simulink model "sim_nomal_regulator"  (R2019a)
settings: Solver=FixedStepAuto  StartTime=0.0  StopTime=20  FixedStep=sT  RelTol=1e-3
InitFcn:
  | sim_param;
values from neighbouring files (symbols this model uses):
  bn = 50    [robot_param.m]    (also in sim_robot_param.m)
  bt = 50    [robot_param.m]    (also in sim_robot_param.m)
  foot_x = 0.07    [robot_param.m]    (also in sim_robot_param.m)
  foot_y = 0.045    [robot_param.m]    (also in sim_robot_param.m)
  foot_z = 0.01    [robot_param.m]    (also in sim_robot_param.m)
  height_plane = 0.025    [robot_param.m]    (also in sim_robot_param.m)
  inix = [0.00 0.00]'    [param.m]    (also in sim_param.m)
  iniXzmax = 0.05    [param.m]    (also in sim_param.m)
  iniXzmin = -0.05    [param.m]    (also in sim_param.m)
  iniy = [0.00 0.00]'    [param.m]    (also in sim_param.m)
  iniYzmax = 0.0625    [param.m]    (also in sim_param.m)
  iniYzmin = -0.0625    [param.m]    (also in sim_param.m)
  kn = 5000    [robot_param.m]    (also in sim_robot_param.m)
  kt = 5000    [robot_param.m]    (also in sim_robot_param.m)
  mu_d = 0.8    [robot_param.m]    (also in sim_robot_param.m)
  mu_s = 2    [robot_param.m]    (also in sim_robot_param.m)
  plane_x = 3    [robot_param.m]    (also in sim_robot_param.m = 6)
  plane_y = 1    [robot_param.m]    (also in sim_robot_param.m)
  R = 20    [param.m]    (also in sim_param.m = 1)
  sT = 0.02    [param.m]    (also in sim_param.m = 0.001)
  torso_offset_x = 0.0    (= 0)    [robot_param.m]    (also in sim_robot_param.m)
  torso_offset_z = -torso_z/2    (= -0.05)    [robot_param.m]    (also in sim_robot_param.m)
  torso_x = 0.1    [robot_param.m]    (also in sim_robot_param.m)
  torso_y = 0.08    [robot_param.m]    (also in sim_robot_param.m)
  torso_z = 0.10    (= 0.1)    [robot_param.m]    (also in sim_robot_param.m)
  w = sqrt(g/zc)    [param.m]    (also in sim_param.m)
  zvt = 1e-3    (= 0.001)    [robot_param.m]    (also in sim_robot_param.m)
undefined symbols (not defined in the file or in its folder): Ad, Bd, Cd, Dd, DiscIntNeverNeededParam, Discrete, sigbuilder_block, Time, X, Y, Z
libraries: nesl_utility x142, sm_lib x86, cstblocks x11, ctrlSharedLib x8
(part 6 of 6)

== stateflow chart sim_nomal_regulator/simulation/Robot/Right Leg/Subsystem4/Chart ==
  state No_Contact/
    (default) -> (junction 3) : {
        | mode = 1;
        |
        | Fn = 0;
        | Fx = 0; Fy = 0;
        | }
  state Sticking
    Sticking -> (junction 35) [order 1] : {
        | Fn = -(kn*pn+bn*dpn);
        | }
    (default) -> (junction 33) : {
        | mode = 4;
        |
        | Fn = -(kn*pn+bn*dpn);
        | }
    (junction 33) -> (junction 35)
    (junction 35) -> (junction 36) [order 1] : [Fn < 0]
    (junction 35) -> (junction 37) [order 2] : {
        | Fx = -(kt*(px-ax)+bt*dpx);
        | Fy = -(kt*(py-ay)+bt*dpy);
        |
        | norm_Ft = sqrt(Fx^2+Fy^2);
        | }
    (junction 36) -> (junction 41) : {
        | mode = 6;
        |
        | Fn = 0;
        | Fx = 0; Fy = 0;
        | }
    (junction 37) -> (junction 40) [order 1] : [norm_Ft > mu_s*Fn]
    (junction 37) -> (junction 38) [order 2]
    (junction 40) -> (junction 42) : {
        | mode = 5;
        |
        | Fx = mu_s*Fn*Fx/norm_Ft;
        | Fy = mu_s*Fn*Fy/norm_Ft;
        | }
    (junction 42) -> (junction 38)
    (junction 41) -> (junction 42)
    (junction 38) -> (junction 39)
  state Sliding
    Sliding -> (junction 10) [order 1] : {
        | mode = 2;
        |
        | Fn = -(kn*pn+bn*dpn);
        | }
    (default) -> (junction 8) : {
        | mode = 2;
        |
        | Fn = -(kn*pn+bn*dpn);
        | }
    (junction 8) -> (junction 10)
    (junction 10) -> (junction 11) [order 1] : [Fn < 0]
    (junction 10) -> (junction 12) [order 2] : {
        | norm_dpt = sqrt(dpx^2+dpy^2);
        | }
    (junction 11) -> (junction 17) : {
        | mode = 6;
        |
        | Fn = 0;
        | Fx = 0; Fy = 0;
        | }
    (junction 12) -> (junction 15) [order 1] : [norm_dpt <= zvt]
    (junction 12) -> (junction 13) [order 2] : {
        | Fx = -mu_d*Fn*dpx/norm_dpt;
        | Fy = -mu_d*Fn*dpy/norm_dpt;
        | }
    (junction 15) -> (junction 16) : {
        | mode = 3;
        | Fx = -mu_d*Fn*dpx/zvt;
        | Fy = -mu_d*Fn*dpy/zvt;
        |
        | ax = px;
        | ay = py;
        | }
    (junction 16) -> (junction 13)
    (junction 17) -> (junction 16)
    (junction 13) -> (junction 14)
  (default) -> No_Contact
  No_Contact -> Sliding : [pn < 0]
  Sliding -> No_Contact [order 1] : [pn >= 0]
  Sticking -> No_Contact [order 1] : [pn >= 0]
  Sliding -> Sticking [order 2] : [pn < 0 ...
      | && mode == 3]
  Sticking -> Sliding [order 2] : [pn < 0 ...
      | && (mode == 5 || mode == 6)]
  data: kn input; kt input; Fx output double; Fy output double; ax local double; ay local double; bn input; bt input; mu_d input; mu_s input; zvt input; px input; py input; pn input; dpx input; dpy input; dpn input; norm_Ft local double; norm_dpt local double; Fn output double; mode output double

== matlab function sim_nomal_regulator/calcULINK ==
  settings: updateMethod=DISCRETE
  data: sT input; u input; sys output; uLINK data_store_memory
function sys = calcULINK(sT,u)

    %u[腰X 腰Y 右足X 右足Y 右足Z 左足X 左足Y 左足Z]

    global uLINK;
    
    persistent cnt;
    if isempty(cnt)
        cnt = 0.0;
    end
    
    ToDeg = 180/pi;
    ToRad = pi/180;
    
    sys = zeros(12,1);
    
    %%% ZMPの計算
    %com = calcCoM;  % 重心位置
    %P = calcP(1);   % 並進運動量
    %L = calcL(1);   % 原点回りの角運動量
    
    %Zc  = com(3);      % 線形倒立振子の設定高さ
    %Tc  = sqrt(Zc/G);  % 線形倒立振子の時定数
    %cx0 = com(1);
    %cy0 = com(2);
    
    
    p0 = uLINK(JointName.BODY).p;
    uLINK(JointName.BODY).p = [u(1), u(2), uLINK(JointName.BODY).p(3)]';
    v = (uLINK(JointName.BODY).p-p0)/sT;
    uLINK(JointName.BODY).v = [v(1) v(2) v(3)]';
    uLINK(JointName.BODY).R = RPY2R([0 0*ToRad 0]);

    %ForwardKinematics(1);
    
    p = [u(3) u(4) u(5)]';
    Rfoot.p = [u(3) u(4) u(5)]';
    Rfoot.R = RPY2R([0 0 0]);
    v = (p-uLINK(JointName.RLEG_FOOT).p)/sT;
    Rfoot.v = [v(1) v(2) v(3)]';
    Rfoot.w = [0 0 0]';
    InverseKinematicsAll(8, Rfoot);
    
    p = [u(6) u(7) u(8)]';
    Lfoot.p = [u(6) u(7) u(8)]';
    Lfoot.R = RPY2R([0 0 0]);
    v = (p-uLINK(JointName.LLEG_FOOT).p)/sT;
    Lfoot.v = [v(1) v(2) v(3)]';
    Lfoot.w = [0 0 0]';
    InverseKinematicsAll(15, Lfoot);
    
    ForwardVelocity(1); 
    
    
    %{
    sys = [90 90 90 90 90 90 90 90 90 90 90 90]';
    
    sys(1) = round(rad2deg(uLINK(JointName.RLEG_J0).q))+90;
    %股関節の剛性不足による胴体の傾き補償フィードフォワード
    sys(2) = round(rad2deg(uLINK(JointName.RLEG_J1).q))+90-0;
    sys(3) = -round(rad2deg(uLINK(JointName.RLEG_J2).q))+90;
    sys(4) = -round(rad2deg(uLINK(JointName.RLEG_J3).q))+90;
    sys(5) = -round(rad2deg(uLINK(JointName.RLEG_J4).q))+90;
    sys(6) = -round(rad2deg(uLINK(JointName.RLEG_J5).q))+90;
    
    sys(7) = round(rad2deg(uLINK(JointName.LLEG_J0).q))+90;
    sys(8) = round(rad2deg(uLINK(JointName.LLEG_J1).q))+90+0;
    sys(9) = -round(rad2deg(uLINK(JointName.LLEG_J2).q))+90;
    sys(10) = -round(rad2deg(uLINK(JointName.LLEG_J3).q))+90;
    sys(11) = -round(rad2deg(uLINK(JointName.LLEG_J4).q))+90;
    sys(12) = -round(rad2deg(uLINK(JointName.LLEG_J5).q))+90;
    %}
    sys(1) = uLINK(JointName.RLEG_J0).q;
    sys(2) = uLINK(JointName.RLEG_J1).q-deg2rad(0);
    sys(3) = uLINK(JointName.RLEG_J2).q;
    sys(4) = uLINK(JointName.RLEG_J3).q;
    sys(5) = uLINK(JointName.RLEG_J4).q;
    sys(6) = uLINK(JointName.RLEG_J5).q;
    sys(7) = uLINK(JointName.LLEG_J0).q;
    sys(8) = uLINK(JointName.LLEG_J1).q+deg2rad(0);
    sys(9) = uLINK(JointName.LLEG_J2).q;
    sys(10) = uLINK(JointName.LLEG_J3).q;
    sys(11) = uLINK(JointName.LLEG_J4).q;
    sys(12) = uLINK(JointName.LLEG_J5).q;
    
    cnt = cnt + sT;
end

== matlab function sim_nomal_regulator/MATLAB Function3 ==
  data: x output; sT input
function x = orbit(sT)

    persistent t; 
    if (isempty(t))     
        t = 0;
    end
    
    %x = zeros(3,1);
    %x = create_orbit(t, 0, 0.6, 0.1);
    x = create_orbit(t, 0, 1.8, 0.3);
    %x = create_orbit(t, 0, 3.0, 0.5);
    
    %{
    x = zeros(3,1);
    if (t > 2)
        x = [0 0.5 0]';
    end
    %}
    t = t + sT;
end

%% 
%
% t:現在時間
% eta0:初期位置
% eta3:最終位置
% d_eta1:最高速度
function Y = create_orbit(t, eta0, eta3, d_eta1)

    %最高速度
    %d_eta1 = 0.1;

    %初期時間
    t0 = 2;
    %加速終了時間（等速度開始時間）
    t1 = 4;
    %等速度終了時間（減速開始時間）
    t2 = 8;
    %減速終了時間
    t3 = 10;


    %加速終了時の位置
    eta1 = eta0 + (d_eta1*(t1-t0)/2);
    %等速終了時の位置
    eta2 = eta1 + (d_eta1*(t2-t1));

    ETA1 = [eta0 0 0 eta1 d_eta1 0]';
    ETA3 = [eta2 d_eta1 0 eta3 0 0]';

    H = [t0^5 t0^4 t0^3 t0^2 t0 1;
        5*t0^4 4*t0^3 3*t0^2 2*t0 1 0;
        20*t0^3 12*t0^2 6*t0 2 0 0;
        t1^5 t1^4 t1^3 t1^2 t1 1;
        5*t1^4 4*t1^3 3*t1^2 2*t1 1 0;
        20*t1^3 12*t1^2 6*t1 2 0 0];
    A = H\ETA1;

    H = [t2^5 t2^4 t2^3 t2^2 t2 1;
        5*t2^4 4*t2^3 3*t2^2 2*t2 1 0;
        20*t2^3 12*t2^2 6*t2 2 0 0;
        t3^5 t3^4 t3^3 t3^2 t3 1;
        5*t3^4 4*t3^3 3*t3^2 2*t3 1 0;
        20*t3^3 12*t3^2 6*t3 2 0 0];
    B = H\ETA3;


    Y = zeros(3,1);
    if (t < t0) 
        Y(1) = eta0;
        Y(2) = 0;
        Y(3) = 0;
    %加速
    elseif (t0 <= t && t < t1) 
        Y(1) = A(1)*t^5 + A(2)*t^4 + A(3)*t^3 + A(4)*t^2 + A(5)*t + A(6);
        Y(2) = 5*A(1)*t^4 + 4*A(2)*t^3 + 3*A(3)*t^2 + 2*A(4)*t + A(5);
        Y(3) = 20*A(1)*t^3 + 12*A(2)*t^2 + 6*A(3)*t + 2*A(4);
    %等速
    elseif (t1 <= t && t <= t2)
        Y(1) = (t-t1)*d_eta1 + eta1;
        Y(2) = d_eta1;
        Y(3) = 0;
    %減速
    elseif (t2 < t && t <= t3)
        Y(1) = B(1)*t^5 + B(2)*t^4 + B(3)*t^3 + B(4)*t^2 + B(5)*t + B(6);
        Y(2) = 5*B(1)*t^4 + 4*B(2)*t^3 + 3*B(3)*t^2 + 2*B(4)*t + B(5);
        Y(3) = 20*B(1)*t^3 + 12*B(2)*t^2 + 6*B(3)*t + 2*B(4);
    else
        Y(1) = eta3;
        Y(2) = 0;
        Y(3) = 0;
    end


end

== matlab function sim_nomal_regulator/regulator1/MATLAB Function ==
  data: refZmp output; xzArea output; yzArea output; x input; legR output; legL output; y input; w input; iniXzmax input; iniXzmin input; iniYzmax input; iniYzmin input; refVx input
function [refZmp,xzArea,yzArea,legR,legL] = fcn(x,y,w,iniXzmax,iniXzmin,iniYzmax,iniYzmin,refVx)
    
    
    %% x軸
    qx = 0.5;
    persistent xR;
    if isempty(xR)
        xR = 0.0;
    end
    persistent xL;
    if isempty(xL)
        xL = 0.0;
    end
    
    %% y軸
    qy = 0.5;
    %r 振幅
    r = 0.05;
    k = 1;
    persistent rho;
    if isempty(rho)
        rho = 1;
    end
    
    %% z軸
    %左足裏内側縁
    xLin = 0.0175;
    %右足裏内側縁
    xRin = -0.0175;
    
    %% y軸
    refy = 0.0;
    zeta = sqrt( (y(1)-refy)^2 + (y(2)^2/(w^2*qy)) );
    f = 1-rho*exp( k*(1-((qy+1)^2*zeta^2)/r^2) );
    yz = refy+(qy+1)*(y(1)-refy + f*(y(2)/w));
    
    yzmax = iniYzmax;
    yzmin = iniYzmin;
    Yz = yz -refy;
    
    %% z軸   
    %右足高さ
    zR = clac(Yz,y,w,rho,xLin,r);
    if (zR > 0) 
        yzmin = refy + xLin;
    end
    %左足高さ
    zL = clac(Yz,y,w,rho,xRin,r);
    if (zL > 0) 
        yzmax = refy + xRin;
    end
    
    if (yz > yzmax)
        yz = yzmax;
    elseif (yz < yzmin)
        yz = yzmin;
    end
    
    refys = y(1)+(y(2)/w);
    yR = -0.04;
    yL = 0.04;
    
    %% x軸
    refx = x(1);
    if (refVx == 0) 
        %立位可安定
        qx = 1.0;
    else
        %速度追従
        qx = 0.0;
    end
    
    %ZMP
    xz = refx+(qx+1)*(x(1)-refx + (x(2)-refVx)/w);
    %着地位置
    refxs = x(1)+(x(2)/w);
    
    if (zR > 0)
        xR = refxs;
        xzmax = xL + iniXzmax;
        xzmin = xL + iniXzmin;
    elseif (zL > 0)
        xL = refxs;
        xzmax = xR + iniXzmax;
        xzmin = xR + iniXzmin;
    else
        if (xL > xR)
            xzmax = xL + iniXzmax;
            xzmin = xR + iniXzmin;
        else
            xzmax = xR + iniXzmax;
            xzmin = xL + iniXzmin;
        end
    end
    
    if (xz > xzmax)
        xz = xzmax;
    elseif (xz < xzmin)
        xz = xzmin;
    end
    
    refZmp = zeros(2,1);
    refZmp = [xz yz]';
    %refZmp = [0 0]';
    xzArea = [xzmax xzmin]';
    yzArea = [yzmax yzmin]';
    
    legR = [xR yR zR]';
    legL = [xL yL zL]';
   
    
end

%% 
function z = clac(yz,x,w,rho,xLin,r)
    
    q = 0.5;
    h = 0.02;
     
    pz = yz - ((q+1)*x(2)/w*sqrt(q))*1i;
    
    %軸足内側に入った
    pLin = xLin - sqrt(complex(abs(pz)^2-xLin^2))*1i;
    %軸足内側から出た
    pLout = xLin + sqrt(complex(abs(pz)^2-xLin^2))*1i;
    
    z = 0;
    phiL = 0;
    %左が軸足
    if (xLin > 0)
        %ZMPが左足にある
        if (real(pz) > xLin)
            %plinからpzまでの角度
            ang_pz = angle(pz)-angle(pLin);
            %pLinからpLoutまでの角度
            ang_io = angle(pLout)-angle(pLin);
            phiL = ang_pz/ang_io;
        end
    %右が軸足
    else
        %ZMPが右足にある
        if (real(pz) < xLin)
            %plinからpzまでの角度（負なので正（第一、第二象限）に移す）
            ang_pz = 0;
            if (angle(pz) > 0) 
                ang_pz = angle(pz)-pi+angle(pLin)+pi; 
            else
                ang_pz = angle(pz)+pi+angle(pLin)+pi; 
            end
            %pLinからpLoutまでの角度（負なので正（第一、第二象限）に移す）
            ang_io = angle(pLin)+pi-angle(pLout)+pi;
            phiL = ang_pz/ang_io;
        end
    end
    
    if (0 < phiL && phiL < 1)
        z = (1/2)*(h*abs(pz)/r)*sigma(rho)*(1-cos(2*pi*phiL));
    end
end

function y = sigma(rho)
    
    if (rho > 1)
        y = 1;
    elseif (exp(-1) <= rho && rho <= 1)
        y = (rho-exp(-1))/(1-exp(-1));
    else
        y = 0;
    end
end

== matlab function sim_nomal_regulator/MATLAB Function1 ==
  settings: updateMethod=DISCRETE
  data: u input; px output; py output; rx input; lx input
function [px,py] = fcn(u,rx,lx)
    
    r = -0.04;
    l = 0.04;
    xs = 0.07/2;
    ys = 0.045/2;
    
    
    r1x = (rx+xs)*u(1);
    r2x = (rx+xs)*u(2);
    r3x = (rx-xs)*u(3);
    r4x = (rx-xs)*u(4);
    PrxfRz = r1x+r2x+r3x+r4x;
    
    r1y = (r+ys)*u(1);
    r2y = (r-ys)*u(2);
    r3y = (r+ys)*u(3);
    r4y = (r-ys)*u(4);
    PryfRz = r1y+r2y+r3y+r4y;
    
    l1x = (lx+xs)*u(5);
    l2x = (lx+xs)*u(6);
    l3x = (lx-xs)*u(7);
    l4x = (lx-xs)*u(8);
    PlxfLz = l1x+l2x+l3x+l4x;
    
    l1y = (l+ys)*u(5);
    l2y = (l-ys)*u(6);
    l3y = (l+ys)*u(7);
    l4y = (l-ys)*u(8);
    PlyfLz = l1y+l2y+l3y+l4y;
    
    fRz = u(1)+u(2)+u(3)+u(4);
    fLz = u(5)+u(6)+u(7)+u(8);
    
    %両足が浮いてない
    if (fRz+fLz ~= 0) 
        %x軸のずれ0.02加算
        px = (PrxfRz+PlxfLz)/(fRz+fLz)+0.02;
        py = (PryfRz+PlyfLz)/(fRz+fLz);
    else
        px = 0;
        py = 0;
    end
    
    %{
    FnR_FrontLeft
    FnR_FrontRight
    FnR_RearLeft
    FnR_RearRight
    
    
    FnL_FrontLeft
    FnL_FrontRight
    FnL_RearLeft
    FnL_RearRight
    %}
    
    
end

== stateflow chart sim_nomal_regulator/simulation/Robot/Right Leg/Subsystem7/Chart ==
  state No_Contact/
    (default) -> (junction 3) : {
        | mode = 1;
        |
        | Fn = 0;
        | Fx = 0; Fy = 0;
        | }
  state Sticking
    Sticking -> (junction 35) [order 1] : {
        | Fn = -(kn*pn+bn*dpn);
        | }
    (default) -> (junction 33) : {
        | mode = 4;
        |
        | Fn = -(kn*pn+bn*dpn);
        | }
    (junction 33) -> (junction 35)
    (junction 35) -> (junction 36) [order 1] : [Fn < 0]
    (junction 35) -> (junction 37) [order 2] : {
        | Fx = -(kt*(px-ax)+bt*dpx);
        | Fy = -(kt*(py-ay)+bt*dpy);
        |
        | norm_Ft = sqrt(Fx^2+Fy^2);
        | }
    (junction 36) -> (junction 41) : {
        | mode = 6;
        |
        | Fn = 0;
        | Fx = 0; Fy = 0;
        | }
    (junction 37) -> (junction 40) [order 1] : [norm_Ft > mu_s*Fn]
    (junction 37) -> (junction 38) [order 2]
    (junction 40) -> (junction 42) : {
        | mode = 5;
        |
        | Fx = mu_s*Fn*Fx/norm_Ft;
        | Fy = mu_s*Fn*Fy/norm_Ft;
        | }
    (junction 42) -> (junction 38)
    (junction 41) -> (junction 42)
    (junction 38) -> (junction 39)
  state Sliding
    Sliding -> (junction 10) [order 1] : {
        | mode = 2;
        |
        | Fn = -(kn*pn+bn*dpn);
        | }
    (default) -> (junction 8) : {
        | mode = 2;
        |
        | Fn = -(kn*pn+bn*dpn);
        | }
    (junction 8) -> (junction 10)
    (junction 10) -> (junction 11) [order 1] : [Fn < 0]
    (junction 10) -> (junction 12) [order 2] : {
        | norm_dpt = sqrt(dpx^2+dpy^2);
        | }
    (junction 11) -> (junction 17) : {
        | mode = 6;
        |
        | Fn = 0;
        | Fx = 0; Fy = 0;
        | }
    (junction 12) -> (junction 15) [order 1] : [norm_dpt <= zvt]
    (junction 12) -> (junction 13) [order 2] : {
        | Fx = -mu_d*Fn*dpx/norm_dpt;
        | Fy = -mu_d*Fn*dpy/norm_dpt;
        | }
    (junction 15) -> (junction 16) : {
        | mode = 3;
        | Fx = -mu_d*Fn*dpx/zvt;
        | Fy = -mu_d*Fn*dpy/zvt;
        |
        | ax = px;
        | ay = py;
        | }
    (junction 16) -> (junction 13)
    (junction 17) -> (junction 16)
    (junction 13) -> (junction 14)
  (default) -> No_Contact
  No_Contact -> Sliding : [pn < 0]
  Sliding -> No_Contact [order 1] : [pn >= 0]
  Sticking -> No_Contact [order 1] : [pn >= 0]
  Sliding -> Sticking [order 2] : [pn < 0 ...
      | && mode == 3]
  Sticking -> Sliding [order 2] : [pn < 0 ...
      | && (mode == 5 || mode == 6)]
  data: kn input; kt input; Fx output double; Fy output double; ax local double; ay local double; bn input; bt input; mu_d input; mu_s input; zvt input; px input; py input; pn input; dpx input; dpy input; dpn input; norm_Ft local double; norm_dpt local double; Fn output double; mode output double

== stateflow chart sim_nomal_regulator/simulation/Robot/Right Leg/Subsystem8/Chart ==
  state No_Contact/
    (default) -> (junction 3) : {
        | mode = 1;
        |
        | Fn = 0;
        | Fx = 0; Fy = 0;
        | }
  state Sticking
    Sticking -> (junction 35) [order 1] : {
        | Fn = -(kn*pn+bn*dpn);
        | }
    (default) -> (junction 33) : {
        | mode = 4;
        |
        | Fn = -(kn*pn+bn*dpn);
        | }
    (junction 33) -> (junction 35)
    (junction 35) -> (junction 36) [order 1] : [Fn < 0]
    (junction 35) -> (junction 37) [order 2] : {
        | Fx = -(kt*(px-ax)+bt*dpx);
        | Fy = -(kt*(py-ay)+bt*dpy);
        |
        | norm_Ft = sqrt(Fx^2+Fy^2);
        | }
    (junction 36) -> (junction 41) : {
        | mode = 6;
        |
        | Fn = 0;
        | Fx = 0; Fy = 0;
        | }
    (junction 37) -> (junction 40) [order 1] : [norm_Ft > mu_s*Fn]
    (junction 37) -> (junction 38) [order 2]
    (junction 40) -> (junction 42) : {
        | mode = 5;
        |
        | Fx = mu_s*Fn*Fx/norm_Ft;
        | Fy = mu_s*Fn*Fy/norm_Ft;
        | }
    (junction 42) -> (junction 38)
    (junction 41) -> (junction 42)
    (junction 38) -> (junction 39)
  state Sliding
    Sliding -> (junction 10) [order 1] : {
        | mode = 2;
        |
        | Fn = -(kn*pn+bn*dpn);
        | }
    (default) -> (junction 8) : {
        | mode = 2;
        |
        | Fn = -(kn*pn+bn*dpn);
        | }
    (junction 8) -> (junction 10)
    (junction 10) -> (junction 11) [order 1] : [Fn < 0]
    (junction 10) -> (junction 12) [order 2] : {
        | norm_dpt = sqrt(dpx^2+dpy^2);
        | }
    (junction 11) -> (junction 17) : {
        | mode = 6;
        |
        | Fn = 0;
        | Fx = 0; Fy = 0;
        | }
    (junction 12) -> (junction 15) [order 1] : [norm_dpt <= zvt]
    (junction 12) -> (junction 13) [order 2] : {
        | Fx = -mu_d*Fn*dpx/norm_dpt;
        | Fy = -mu_d*Fn*dpy/norm_dpt;
        | }
    (junction 15) -> (junction 16) : {
        | mode = 3;
        | Fx = -mu_d*Fn*dpx/zvt;
        | Fy = -mu_d*Fn*dpy/zvt;
        |
        | ax = px;
        | ay = py;
        | }
    (junction 16) -> (junction 13)
    (junction 17) -> (junction 16)
    (junction 13) -> (junction 14)
  (default) -> No_Contact
  No_Contact -> Sliding : [pn < 0]
  Sliding -> No_Contact [order 1] : [pn >= 0]
  Sticking -> No_Contact [order 1] : [pn >= 0]
  Sliding -> Sticking [order 2] : [pn < 0 ...
      | && mode == 3]
  Sticking -> Sliding [order 2] : [pn < 0 ...
      | && (mode == 5 || mode == 6)]
  data: kn input; kt input; Fx output double; Fy output double; ax local double; ay local double; bn input; bt input; mu_d input; mu_s input; zvt input; px input; py input; pn input; dpx input; dpy input; dpn input; norm_Ft local double; norm_dpt local double; Fn output double; mode output double

== stateflow chart sim_nomal_regulator/simulation/Robot/Right Leg/Subsystem9/Chart ==
  state No_Contact/
    (default) -> (junction 3) : {
        | mode = 1;
        |
        | Fn = 0;
        | Fx = 0; Fy = 0;
        | }
  state Sticking
    Sticking -> (junction 35) [order 1] : {
        | Fn = -(kn*pn+bn*dpn);
        | }
    (default) -> (junction 33) : {
        | mode = 4;
        |
        | Fn = -(kn*pn+bn*dpn);
        | }
    (junction 33) -> (junction 35)
    (junction 35) -> (junction 36) [order 1] : [Fn < 0]
    (junction 35) -> (junction 37) [order 2] : {
        | Fx = -(kt*(px-ax)+bt*dpx);
        | Fy = -(kt*(py-ay)+bt*dpy);
        |
        | norm_Ft = sqrt(Fx^2+Fy^2);
        | }
    (junction 36) -> (junction 41) : {
        | mode = 6;
        |
        | Fn = 0;
        | Fx = 0; Fy = 0;
        | }
    (junction 37) -> (junction 40) [order 1] : [norm_Ft > mu_s*Fn]
    (junction 37) -> (junction 38) [order 2]
    (junction 40) -> (junction 42) : {
        | mode = 5;
        |
        | Fx = mu_s*Fn*Fx/norm_Ft;
        | Fy = mu_s*Fn*Fy/norm_Ft;
        | }
    (junction 42) -> (junction 38)
    (junction 41) -> (junction 42)
    (junction 38) -> (junction 39)
  state Sliding
    Sliding -> (junction 10) [order 1] : {
        | mode = 2;
        |
        | Fn = -(kn*pn+bn*dpn);
        | }
    (default) -> (junction 8) : {
        | mode = 2;
        |
        | Fn = -(kn*pn+bn*dpn);
        | }
    (junction 8) -> (junction 10)
    (junction 10) -> (junction 11) [order 1] : [Fn < 0]
    (junction 10) -> (junction 12) [order 2] : {
        | norm_dpt = sqrt(dpx^2+dpy^2);
        | }
    (junction 11) -> (junction 17) : {
        | mode = 6;
        |
        | Fn = 0;
        | Fx = 0; Fy = 0;
        | }
    (junction 12) -> (junction 15) [order 1] : [norm_dpt <= zvt]
    (junction 12) -> (junction 13) [order 2] : {
        | Fx = -mu_d*Fn*dpx/norm_dpt;
        | Fy = -mu_d*Fn*dpy/norm_dpt;
        | }
    (junction 15) -> (junction 16) : {
        | mode = 3;
        | Fx = -mu_d*Fn*dpx/zvt;
        | Fy = -mu_d*Fn*dpy/zvt;
        |
        | ax = px;
        | ay = py;
        | }
    (junction 16) -> (junction 13)
    (junction 17) -> (junction 16)
    (junction 13) -> (junction 14)
  (default) -> No_Contact
  No_Contact -> Sliding : [pn < 0]
  Sliding -> No_Contact [order 1] : [pn >= 0]
  Sticking -> No_Contact [order 1] : [pn >= 0]
  Sliding -> Sticking [order 2] : [pn < 0 ...
      | && mode == 3]
  Sticking -> Sliding [order 2] : [pn < 0 ...
      | && (mode == 5 || mode == 6)]
  data: kn input; kt input; Fx output double; Fy output double; ax local double; ay local double; bn input; bt input; mu_d input; mu_s input; zvt input; px input; py input; pn input; dpx input; dpy input; dpn input; norm_Ft local double; norm_dpt local double; Fn output double; mode output double
